simulink model "plant_test"  (R2021a)
settings: Solver=VariableStepAuto  StartTime=0.0  StopTime=10  MaxStep=0.01  RelTol=1e-3
values from neighbouring files (symbols this model uses):
  b_PID_hoist = -MEh * nh * wh    (= -542577.777778)    [Data.m]
  b_PID_trolley = MEtd*ntd*wtd    (= 540180)    [Data.m]
  bEh = 2*(bhd + bhm*ih^2)/rhd^2    (= 31004.4444444)    [Data.m]
  bEtd = (btd + btm*it^2)/rtd^2    (= 21607.2)    [Data.m]
  bt = 90    [Data.m]
  btw = 3e6    (= 3000000)    [Data.m]
  g = 9.80665    [Data.m]
  hoist_brake = readValue(uaClient,hoist_brake_node)    [Level1_OPC.m]    (also in test__TLK.m = 1; test_hoist.m = 0; test_trolley.m = 1)
  hoist_ebrake = readValue(uaClient,hoist_ebrake_node)    [Level1_OPC.m]    (also in test__TLK.m = 0; test_hoist.m = 0; test_trolley.m = 1)
  ih = 22    [Data.m]
  it = 30    [Data.m]
  Ksa_PID_hoist = -MEh * nh * wh^2    (= -1807802.81417)    [Data.m]
  Ksa_PID_trolley = MEtd*ntd*wtd^2    (= 3890592.432)    [Data.m]
  Ksia_PID_hoist = -MEh * nh * wh^3    (= -6023377.93542)    [Data.m]
  Ksia_PID_trolley = MEtd*ntd*wtd^3    (= 28021602.9322)    [Data.m]
  lh0 = 45 + 9.35    (= 54.35)    [test__TLK.m]    (also in test_hoist.m = 20; test_trolley.m = 10)
  MEh = 2*(Jhd_hEb + Jhm_hb * ih^2)/rhd^2    (= 65137.7777778)    [Data.m]
  MEtd = (Jtd + Jtm_tb*it^2)/rtd^2    (= 30000)    [Data.m]
  Ms = 15000    [Data.m]
  Mt = 30000    [Data.m]
  rhd = 0.75    [Data.m]
  rtd = 0.5    [Data.m]
  Tau_hm = 1e-3    (= 0.001)    [Data.m]
  Tau_tm = 1e-3    (= 0.001)    [Data.m]
  Th = 0    [test__TLK.m]    (also in test_hoist.m = Thm_max/5; test_trolley.m)
  Thm_max = 2.0e4    (= 20000)    [Data.m]
  trolley_brake = readValue(uaClient,trolley_brake_node)    [Level1_OPC.m]    (also in test__TLK.m = 0; test_hoist.m = 0; test_trolley.m = 0)
  Tt = 0    [test__TLK.m]    (also in test_hoist.m; test_trolley.m = Ttm_max/2)
  Ttm_max = 3.0e3    (= 3000)    [Data.m]
  xt0 = 10.55    [test__TLK.m]    (also in test_hoist.m = -20; test_trolley.m = -25)
  xtd0 = 10.55    [test__TLK.m]    (also in test_hoist.m = -20; test_trolley.m = -25)
  Yt0 = 45    [Data.m]
undefined symbols (not defined in the file or in its folder): sigbuilder_block
libraries: simulink x2
settings Model: Creator=jpss8  LastModifiedBy=jpss8

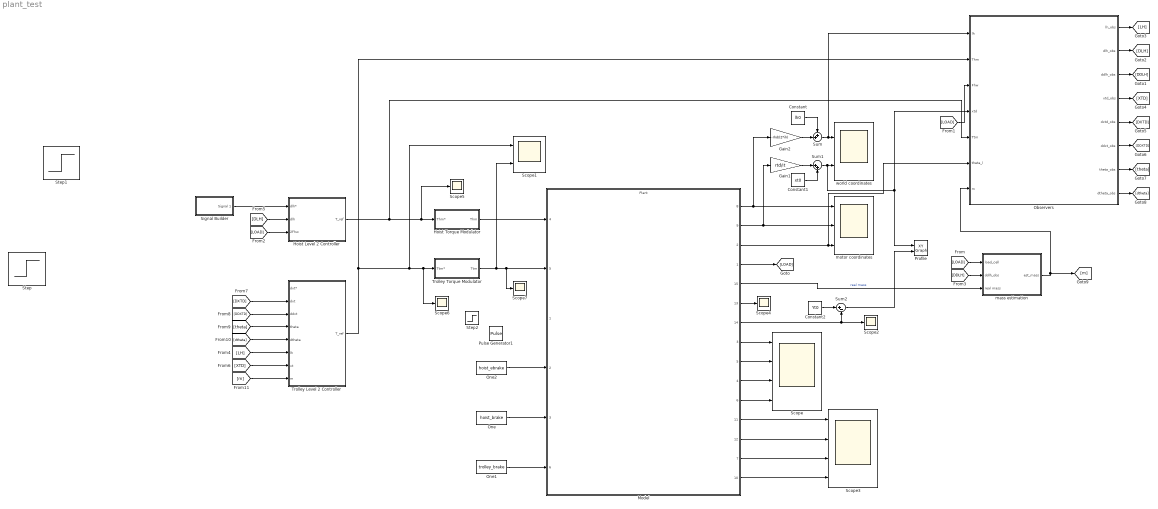
== system plant_test ==
  Constant : Constant  Value=lh0
  Constant1 : Constant  Value=xt0
  Constant2 : Constant  Value=Yt0
  Gain1 : Gain  Gain=rtd/it
  Gain2 : Gain  Gain=-rhd/(2*ih)
  Hoist Level 2 Controller : Subsystem
  Hoist Torque Modulator : Subsystem
  Model : ModelReference  ModelNameDialog=Plant.slx  SimulationMode=Normal  ModelReferenceVersion=1.173
      settings: PortSchema="{\"entries\":[{\"content\":{\"sides\":[{\"content\":{\"connectorIds\":[\"In4\",\"In5\",\"In1\",\"In2\",\"In3\",\"In6\"]},\"type\":\"ConnectorPlacement.EquallySpacedRectSide\",\"uuid\":\"c8db36dc-26e4-465b-ba81-4ad6698d5333\"},{\"content\":{\"connectorIds\":[\"Out8\",\"Out9\",\"Out2\",\"Out1\",\"Out15\",\"Out13\",\"Out14\",\"Out3\",\"Out5\",\"Out4\",\"Out6\",\"Out11\",\"Out12\",\"Out7\",\"Out10\"],\"side\":\"RIGHT\"},\"type\":\"ConnectorPlacement.EquallySpacedRectSide\",\"uuid\":\"9d1fafb8-102d-4671-8cf9-42f2986bdf69\"},{\"content\":{\"connectorIds\":[],\"side\":\"TOP\"},\"type\":\"ConnectorPlacement.EquallySpacedRectSide\",\"uuid\":\"31c48a41-488d-445d-a89d-3c2736ead4dc\"}]},\"type\":\"ConnectorPlacement.EquallySpacedConnector\",\"uuid\":\"271b3c7a-5021-4a95-89d3-3220f33b08df\"}],\"packageUris\":[\"http://schema.mathworks.com/mf0/Connector/R2020b\"],\"version\":\"1.0\"}"
  Observers : Subsystem
  One : Constant  Value=hoist_brake  OutDataTypeStr=Inherit: Inherit via back propagation
  One1 : Constant  Value=trolley_brake  OutDataTypeStr=Inherit: Inherit via back propagation
  One2 : Constant  Value=hoist_ebrake  OutDataTypeStr=Inherit: Inherit via back propagation
  Profile : simulink/Sinks/XY Graph  xmin=-30  xmax=50  ymin=-50  ymax=50  st=-1
  Pulse Generator1 : DiscretePulseGenerator  PulseType=Time based  Period=50  PulseWidth=10  PhaseDelay=1
  Scope : Scope  NumInputPorts=4
  Scope1 : Scope  NumInputPorts=2
  Scope{2,4..7} (5 alike) : Scope
  Scope3 : Scope  NumInputPorts=4
  Signal Builder : Subsystem  Tag=STV Subsys  LoadFcn=sigbuilder_block('load');  StartFcn=sigbuilder_block('start');  StopFcn=sigbuilder_block('stop');  ClipboardFcn=sigbuilder_block('clipboard');  mask(Sigbuilder block){tuvar=[0:10]}
      mask help: Simulink:masks:SigbuilderBlock_MD
      mask init:
      | if ~strcmp(get_param(bdroot(gcbh),'SimulationStatus'),'stopped') tuvar = sigbuilder_block('maskInit'); end
      settings: CopyFcn=sigbuilder_block('copy');  DeleteFcn=sigbuilder_block('delete');  ModelCloseFcn=sigbuilder_block('modelClose');  PreSaveFcn=sigbuilder_block('preSave');  PauseFcn=sigbuilder_block('pause');  ContinueFcn=sigbuilder_block('continue');  NameChangeFcn=sigbuilder_block('namechange');  OpenFcn=sigbuilder_block('open',[437.6 199.2 550.4 400 ]);  CloseFcn=sigbuilder_block('close');
      mask Display: plot(0, 0, 100, 100,[2, 2, 32, 32, 2], [68, 8, 8, 68, 68],[32, 2], [38, 38], [32, 19, 2],[53, 60, 44], [32, 17, 17, 2],[16, 16, 31, 31]);txt = getActiveGroup(gcbh);text(2, 100, txt,'verticalAlignment', 'top');
  Step : Step  After=Tt  SampleTime=0
  Step1 : Step  Time=0.5  After=Th  SampleTime=0
  Step2 : Step  Time=0.25  SampleTime=0
  Sum : Sum  Inputs=++|
  Sum1 : Sum  Inputs=|++
  Sum2 : Sum  Inputs=|+-
  Trolley Level 2 Controller : Subsystem
  Trolley Torque Modulator : Subsystem
  mass estimation : Subsystem
  motor coordinates : Scope  NumInputPorts=3
  world coordinates : Scope  NumInputPorts=2
  wires:
  Trolley Level 2 Controller/1(T_ref) -> Observers/2(Thm), Scope1/1, Scope6/1, Trolley Torque Modulator/1(Ttm*)
  Model/9 -> motor coordinates/2, Gain1/1
  Model/8 -> Gain2/1, motor coordinates/1
  Model/2 -> Observers/6(theta_l), motor coordinates/3
  Model/1 -> [LOAD]
  Model/15 -> mass estimation/3(real mass)  "real mass"
  Gain1/1 -> Sum1/1
  Gain2/1 -> Sum/2
  One1/1 -> Model/6
  One2/1 -> Model/2
  Sum/1 -> Observers/1(lh), world coordinates/1
  Constant/1 -> Sum/1
  Constant1/1 -> Sum1/2
  Model/14 -> Sum2/2, Scope2/1
  Constant2/1 -> Sum2/1
  Sum2/1 -> Profile/2
  Model/3 -> Scope/1
  Model/5 -> Scope/2
  Model/4 -> Scope/3
  Model/6 -> Scope/4
  Model/11 -> Scope3/1
  Model/12 -> Scope3/2
  Model/7 -> Scope3/3
  Model/10 -> Scope3/4
  Model/13 -> Scope4/1
  One/1 -> Model/3
  Sum1/1 -> Observers/4(xtd), Profile/1, world coordinates/2
  mass estimation/1(est_mass) -> [m], Observers/7(m)
  Observers/3(ddlh_obs) -> [DDLH]
  Hoist Torque Modulator/1(Thm) -> Model/4
  Trolley Torque Modulator/1(Ttm) -> Scope1/2, Scope7/1, Model/5
  Hoist Level 2 Controller/1(T_ref) -> Observers/5(Ttm), Scope5/1, Hoist Torque Modulator/1(Thm*)
  [LOAD] -> mass estimation/1(load_cell)
  [LOAD] -> Observers/3(Fhw)
  [LOAD] -> Hoist Level 2 Controller/3(2Fhw)
  [DDLH] -> mass estimation/2(ddlh_obs)
  Observers/2(dlh_obs) -> [DLH]
  Observers/1(lh_obs) -> [LH]
  [DLH] -> Hoist Level 2 Controller/2(dlh)
  Observers/6(ddxt_obs) -> [DDXTD]
  Observers/5(dxtd_obs) -> [DXTD]
  Observers/4(xtd_obs) -> [XTD]
  [DXTD] -> Trolley Level 2 Controller/2(dxt)
  [DDXTD] -> Trolley Level 2 Controller/3(ddxt)
  [LH] -> Trolley Level 2 Controller/6(lh)
  [XTD] -> Trolley Level 2 Controller/7(xt)
  Observers/7(theta_obs) -> [theta]
  Observers/8(dtheta_obs) -> [dtheta]
  [theta] -> Trolley Level 2 Controller/4(theta)
  [dtheta] -> Trolley Level 2 Controller/5(dtheta)
  [m] -> Trolley Level 2 Controller/8(m)
  Signal Builder/1(Signal 1) -> Hoist Level 2 Controller/1(dlh*)

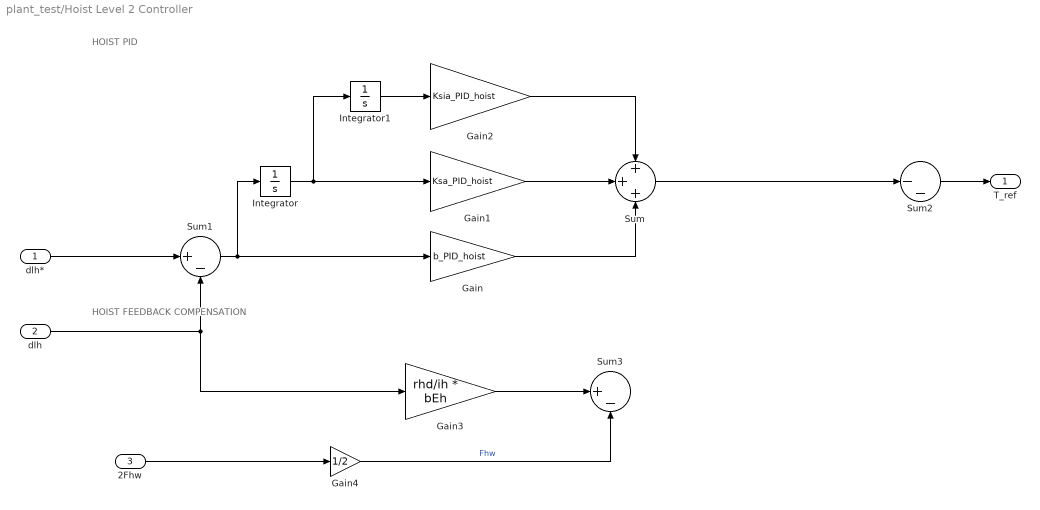
== system plant_test/Hoist Level 2 Controller ==
  note: HOIST FEEDBACK COMPENSATION
  note: HOIST PID
  dlh* : Inport
  dlh : Inport  Port=2
  2Fhw : Inport  Port=3
  Gain : Gain  Gain=b_PID_hoist
  Gain1 : Gain  Gain=Ksa_PID_hoist
  Gain2 : Gain  Gain=Ksia_PID_hoist
  Gain3 : Gain  Gain=rhd/ih * bEh
  Gain4 : Gain  Gain=1/2
  Integrator : Integrator
  Integrator1 : Integrator
  Sum : Sum  Inputs=+++
  Sum1 : Sum  Inputs=|+-
  Sum2 : Sum  Inputs=|--
  Sum3 : Sum  Inputs=|+-
  T_ref : Outport
  wires:
  Integrator/1 -> Integrator1/1, Gain1/1
  Integrator1/1 -> Gain2/1
  Gain1/1 -> Sum/2
  Gain2/1 -> Sum/1
  Gain/1 -> Sum/3
  Sum1/1 -> Gain/1, Integrator/1
  Sum/1 -> Sum2/1
  Gain3/1 -> Sum3/1
  2Fhw/1 -> Gain4/1
  Gain4/1 -> Sum3/2  "Fhw"
  dlh/1 -> Gain3/1, Sum1/2
  dlh*/1 -> Sum1/1
  Sum2/1 -> T_ref/1

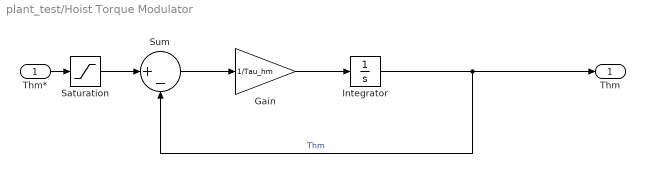
== system plant_test/Hoist Torque Modulator ==
  Thm* : Inport
  Gain : Gain  Gain=1/Tau_hm
  Integrator : Integrator
  Saturation : Saturate  UpperLimit=Thm_max  LowerLimit=-Thm_max
  Sum : Sum  Inputs=|+-
  Thm : Outport
  wires:
  Integrator/1 -> Sum/2, Thm/1  "Thm"
  Sum/1 -> Gain/1
  Gain/1 -> Integrator/1
  Thm*/1 -> Saturation/1
  Saturation/1 -> Sum/1

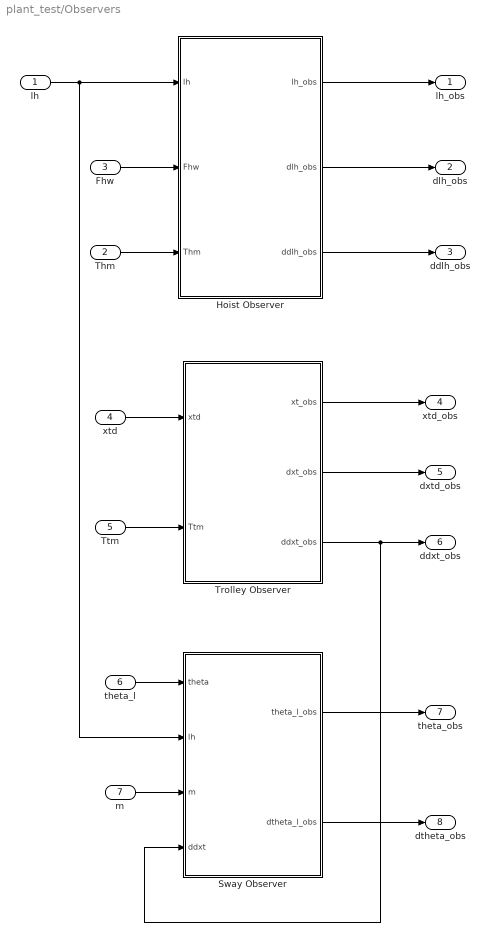
== system plant_test/Observers ==
  lh : Inport
  Thm : Inport  Port=2
  Fhw : Inport  Port=3
  xtd : Inport  Port=4
  Ttm : Inport  Port=5
  theta_l : Inport  Port=6
  m : Inport  Port=7
  Hoist Observer : Subsystem
  Sway Observer : Subsystem
  Trolley Observer : Subsystem
  lh_obs : Outport
  dlh_obs : Outport  Port=2
  ddlh_obs : Outport  Port=3
  xtd_obs : Outport  Port=4
  dxtd_obs : Outport  Port=5
  ddxt_obs : Outport  Port=6
  theta_obs : Outport  Port=7
  dtheta_obs : Outport  Port=8
  wires:
  xtd/1 -> Trolley Observer/1(xtd)
  Ttm/1 -> Trolley Observer/2(Ttm)
  Trolley Observer/1(xt_obs) -> xtd_obs/1
  Trolley Observer/2(dxt_obs) -> dxtd_obs/1
  Fhw/1 -> Hoist Observer/2(Fhw)
  Thm/1 -> Hoist Observer/3(Thm)
  Hoist Observer/1(lh_obs) -> lh_obs/1
  Hoist Observer/2(dlh_obs) -> dlh_obs/1
  theta_l/1 -> Sway Observer/1(theta)
  m/1 -> Sway Observer/3(m)
  Trolley Observer/3(ddxt_obs) -> Sway Observer/4(ddxt), ddxt_obs/1
  lh/1 -> Hoist Observer/1(lh), Sway Observer/2(lh)
  Hoist Observer/3(ddlh_obs) -> ddlh_obs/1
  Sway Observer/1(theta_l_obs) -> theta_obs/1
  Sway Observer/2(dtheta_l_obs) -> dtheta_obs/1

== system plant_test/Signal Builder ==
  Demux : Demux  Tag=STV Demux  Outputs=1
      settings: DisplayOption=none
  FromWs : FromWorkspace  Tag=STV FromWs  VariableName=tuvar
      SigBuilderData=|
      | common.afterFinalStr = 'Extrapolate'
      | common.sampleTime = 0
      | dataSet.timeRange = [0 10]
      | dataSet.name = 'Group 1'
      | sbobj.Groups.Name = 'Group 1'
      | sbobj.Groups.Signals.Name = 'Signal 1'
      | sbobj.Groups.Signals.XData = [0 2 8 10]
      | sbobj.Groups.Signals.YData = [0 3 3 0]
  Signal 1 : Outport  Tag=STV Outport
  wires:
  Demux/1 -> Signal 1/1
  FromWs/1 -> Demux/1

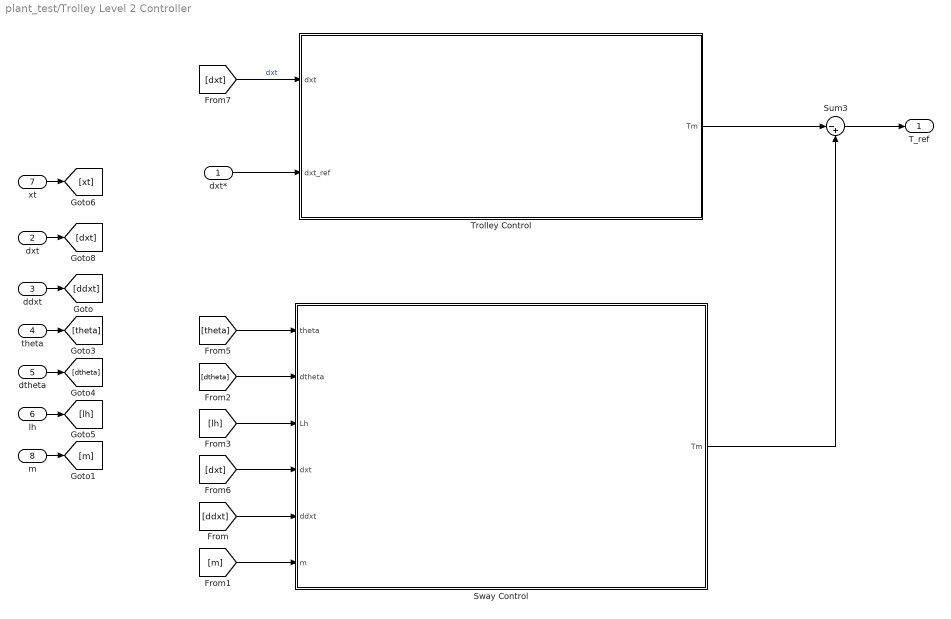
== system plant_test/Trolley Level 2 Controller ==
  dxt* : Inport
  dxt : Inport  Port=2
  ddxt : Inport  Port=3
  theta : Inport  Port=4
  dtheta : Inport  Port=5
  lh : Inport  Port=6
  xt : Inport  Port=7
  m : Inport  Port=8
  Sum3 : Sum  Inputs=|-+
  Sway Control : Subsystem
  Trolley Control : Subsystem
  T_ref : Outport
  wires:
  ddxt/1 -> [ddxt]
  lh/1 -> [lh]
  dtheta/1 -> [dtheta]
  theta/1 -> [theta]
  dxt/1 -> [dxt]
  [dxt] -> Trolley Control/1(dxt)  "dxt"
  Sum3/1 -> T_ref/1
  [lh] -> Sway Control/3(Lh)
  [dxt] -> Sway Control/4(dxt)
  xt/1 -> [xt]
  dxt*/1 -> Trolley Control/2(dxt_ref)
  Sway Control/1(Tm) -> Sum3/2
  [theta] -> Sway Control/1(theta)
  [dtheta] -> Sway Control/2(dtheta)
  Trolley Control/1(Tm) -> Sum3/1
  [ddxt] -> Sway Control/5(ddxt)
  [m] -> Sway Control/6(m)
  m/1 -> [m]

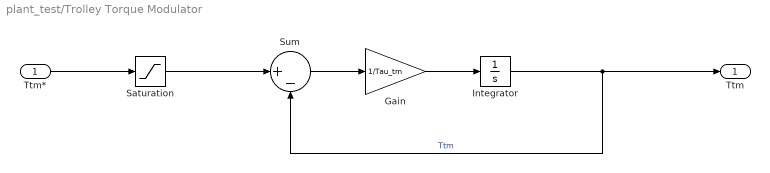
== system plant_test/Trolley Torque Modulator ==
  Ttm* : Inport
  Gain : Gain  Gain=1/Tau_tm
  Integrator : Integrator
  Saturation : Saturate  UpperLimit=Ttm_max  LowerLimit=-Ttm_max
  Sum : Sum  Inputs=|+-
  Ttm : Outport
  wires:
  Gain/1 -> Integrator/1
  Sum/1 -> Gain/1
  Integrator/1 -> Ttm/1, Sum/2  "Ttm"
  Ttm*/1 -> Saturation/1
  Saturation/1 -> Sum/1

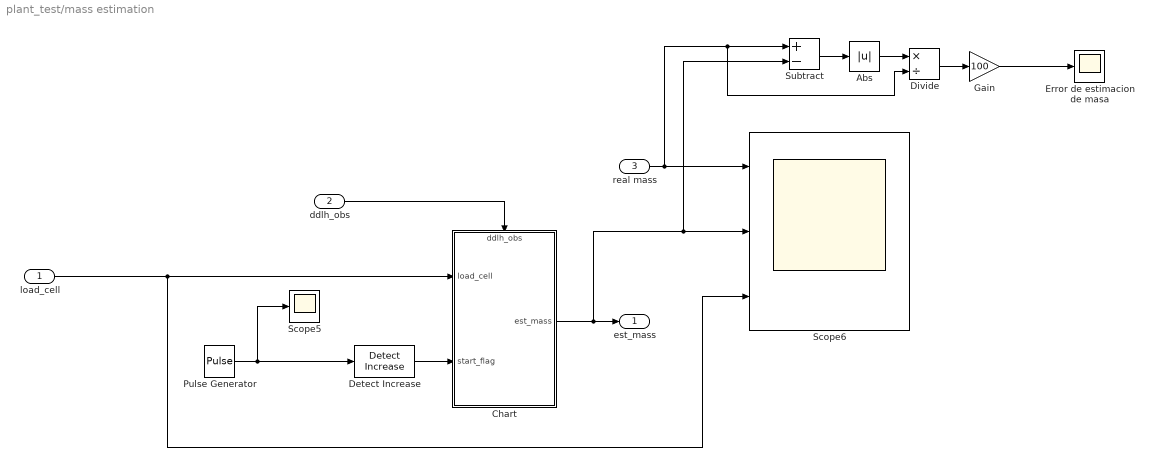
== system plant_test/mass estimation ==
  load_cell : Inport
  ddlh_obs : Inport  Port=2
  real mass : Inport  Port=3
  Abs : Abs
  Chart : Stateflow chart  TreatAsAtomicUnit=on
      settings: PortSchema="{\"entries\":[{\"content\":{\"sides\":[{\"content\":{\"connectorIds\":[\"In2\",\"In3\"]},\"type\":\"ConnectorPlacement.EquallySpacedRectSide\",\"uuid\":\"44794d8c-8d17-4178-a01f-d04d4719ed54\"},{\"content\":{\"connectorIds\":[\"Out1\"],\"side\":\"RIGHT\"},\"type\":\"ConnectorPlacement.EquallySpacedRectSide\",\"uuid\":\"4fbe92f0-b9dd-4e22-a980-5654a9e61553\"},{\"content\":{\"connectorIds\":[\"In1\"],\"side\":\"TOP\"},\"type\":\"ConnectorPlacement.EquallySpacedRectSide\",\"uuid\":\"c0e4bb71-f4b3-4ee0-bf7e-beab745a0d9c\"}]},\"type\":\"ConnectorPlacement.EquallySpacedConnector\",\"uuid\":\"86c94122-6cae-4719-99cd-dfe2bbeee74d\"}],\"packageUris\":[\"http://schema.mathworks.com/mf0/Connector/R2020b\"],\"version\":\"1.0\"}"
  Detect Increase : simulink/Logic and Bit Operations/Detect Increase  vinit=0.0  OutDataTypeStr=boolean
  Divide : Product  Inputs=*/
  Error de estimacion de masa : Scope
  Gain : Gain  Gain=100
  Pulse Generator : DiscretePulseGenerator  PulseType=Time based  Period=50  PulseWidth=2  PhaseDelay=3
  Scope5 : Scope
  Scope6 : Scope  NumInputPorts=3
  Subtract : Sum  Inputs=+-
  est_mass : Outport
  wires:
  load_cell/1 -> Chart/2(load_cell), Scope6/3
  Detect Increase/1 -> Chart/3(start_flag)
  Pulse Generator/1 -> Scope5/1, Detect Increase/1
  Chart/1(est_mass) -> est_mass/1, Subtract/2, Scope6/2
  real mass/1 -> Divide/2, Subtract/1, Scope6/1
  Subtract/1 -> Abs/1
  Abs/1 -> Divide/1
  Divide/1 -> Gain/1
  Gain/1 -> Error de estimacion de masa/1
  ddlh_obs/1 -> Chart/1(ddlh_obs)

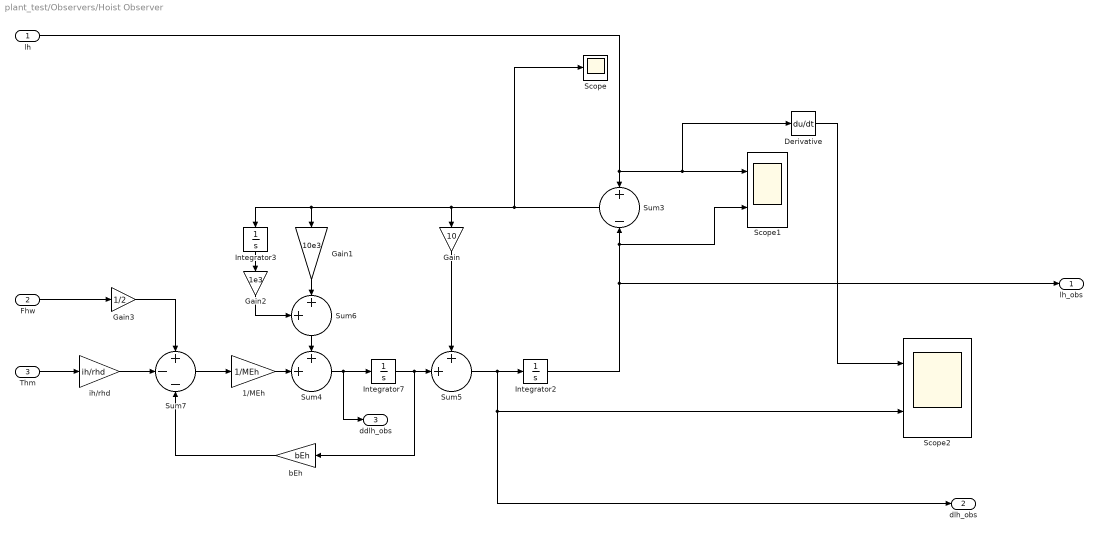
== system plant_test/Observers/Hoist Observer ==
  lh : Inport
  Fhw : Inport  Port=2
  Thm : Inport  Port=3
  1/MEh : Gain  Gain=1/MEh
  Derivative : Derivative
  Gain : Gain  Gain=10
  Gain1 : Gain  Gain=10e3
  Gain2 : Gain  Gain=1e3
  Gain3 : Gain  Gain=1/2
  Integrator2 : Integrator  InitialCondition=lh0
  Integrator3 : Integrator
  Integrator7 : Integrator
  Scope : Scope
  Scope1 : Scope  NumInputPorts=2
  Scope2 : Scope  NumInputPorts=2
  Sum3 : Sum  Inputs=+|-
  Sum4 : Sum  Inputs=++|
  Sum5 : Sum  Inputs=++|
  Sum6 : Sum  Inputs=++|
  Sum7 : Sum  Inputs=+--
  bEh : Gain  Gain=bEh
  ih/rhd : Gain  Gain=ih/rhd
  lh_obs : Outport
  dlh_obs : Outport  Port=2
  ddlh_obs : Outport  Port=3
  wires:
  Sum5/1 -> dlh_obs/1, Scope2/2, Integrator2/1
  lh/1 -> Sum3/1, Derivative/1, Scope1/1
  Gain1/1 -> Sum6/2
  Gain3/1 -> Sum7/1
  Integrator3/1 -> Gain2/1
  bEh/1 -> Sum7/3
  Sum3/1 -> Scope/1, Gain/1, Integrator3/1, Gain1/1
  ih/rhd/1 -> Sum7/2
  Sum7/1 -> 1/MEh/1
  Sum4/1 -> ddlh_obs/1, Integrator7/1
  Gain/1 -> Sum5/1
  Integrator2/1 -> lh_obs/1, Scope1/2, Sum3/2
  Sum6/1 -> Sum4/1
  Integrator7/1 -> bEh/1, Sum5/2
  1/MEh/1 -> Sum4/2
  Derivative/1 -> Scope2/1
  Thm/1 -> ih/rhd/1
  Fhw/1 -> Gain3/1
  Gain2/1 -> Sum6/1

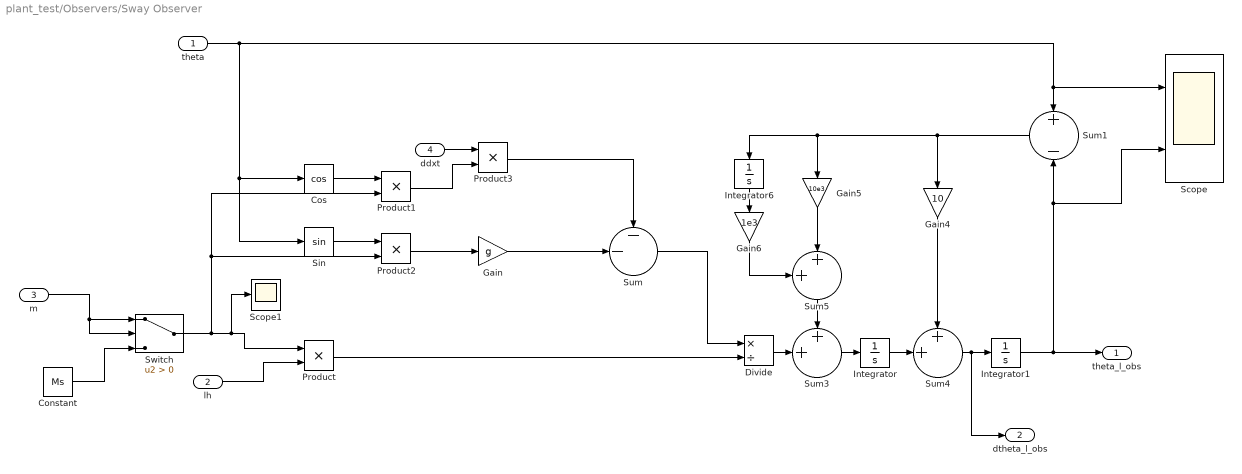
== system plant_test/Observers/Sway Observer ==
  theta : Inport
  lh : Inport  Port=2
  m : Inport  Port=3
  ddxt : Inport  Port=4
  Constant : Constant  Value=Ms
  Cos : Trigonometry  Operator=cos
  Divide : Product  Inputs=*/
  Gain : Gain  Gain=g
  Gain4 : Gain  Gain=10
  Gain5 : Gain  Gain=10e3
  Gain6 : Gain  Gain=1e3
  Integrator : Integrator
  Integrator1 : Integrator
  Integrator6 : Integrator
  Product{,1..3} (4 alike) : Product
  Scope : Scope  NumInputPorts=2
  Scope1 : Scope
  Sin : Trigonometry
  Sum : Sum  Inputs=--|
  Sum1 : Sum  Inputs=+|-
  Sum3 : Sum  Inputs=++|
  Sum4 : Sum  Inputs=++|
  Sum5 : Sum  Inputs=++|
  Switch : Switch  Criteria=u2 > Threshold
  theta_l_obs : Outport
  dtheta_l_obs : Outport  Port=2
  wires:
  Product/1 -> Divide/2
  theta/1 -> Sin/1, Cos/1, Scope/1, Sum1/1
  lh/1 -> Product/2
  Divide/1 -> Sum3/2
  Product3/1 -> Sum/1
  Cos/1 -> Product1/1
  Sin/1 -> Product2/1
  Product2/1 -> Gain/1
  Gain/1 -> Sum/2
  Product1/1 -> Product3/2
  ddxt/1 -> Product3/1
  Sum/1 -> Divide/1
  Integrator1/1 -> theta_l_obs/1, Scope/2, Sum1/2
  Sum1/1 -> Gain5/1, Integrator6/1, Gain4/1
  Gain5/1 -> Sum5/2
  Integrator6/1 -> Gain6/1
  Gain6/1 -> Sum5/1
  Sum3/1 -> Integrator/1
  Sum4/1 -> dtheta_l_obs/1, Integrator1/1
  Sum5/1 -> Sum3/1
  Gain4/1 -> Sum4/1
  Integrator/1 -> Sum4/2
  m/1 -> Switch/2, Switch/1
  Switch/1 -> Scope1/1, Product/1, Product1/2, Product2/2
  Constant/1 -> Switch/3

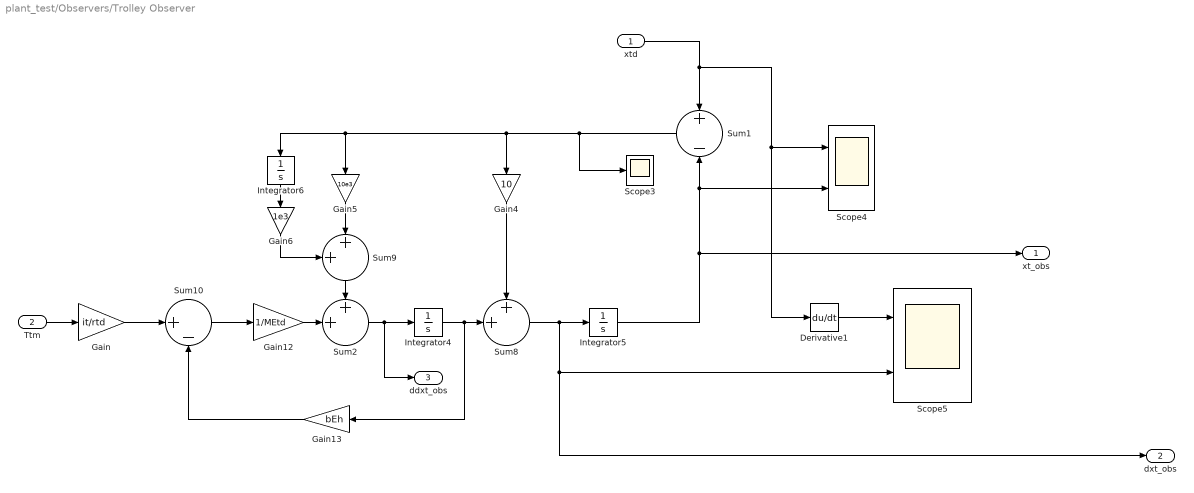
== system plant_test/Observers/Trolley Observer ==
  xtd : Inport
  Ttm : Inport  Port=2
  Derivative1 : Derivative
  Gain : Gain  Gain=it/rtd
  Gain12 : Gain  Gain=1/MEtd
  Gain13 : Gain  Gain=bEh
  Gain4 : Gain  Gain=10
  Gain5 : Gain  Gain=10e3
  Gain6 : Gain  Gain=1e3
  Integrator4 : Integrator
  Integrator5 : Integrator  InitialCondition=xtd0
  Integrator6 : Integrator
  Scope3 : Scope
  Scope4 : Scope  NumInputPorts=2
  Scope5 : Scope  NumInputPorts=2
  Sum1 : Sum  Inputs=+|-
  Sum10 : Sum  Inputs=|+-
  Sum2 : Sum  Inputs=++|
  Sum8 : Sum  Inputs=++|
  Sum9 : Sum  Inputs=++|
  xt_obs : Outport
  dxt_obs : Outport  Port=2
  ddxt_obs : Outport  Port=3
  wires:
  Sum2/1 -> ddxt_obs/1, Integrator4/1
  Sum8/1 -> Integrator5/1, dxt_obs/1, Scope5/2
  Gain4/1 -> Sum8/1
  Integrator4/1 -> Sum8/2, Gain13/1
  Sum1/1 -> Gain5/1, Integrator6/1, Gain4/1, Scope3/1
  Derivative1/1 -> Scope5/1
  Integrator5/1 -> xt_obs/1, Sum1/2, Scope4/2
  xtd/1 -> Sum1/1, Derivative1/1, Scope4/1
  Gain12/1 -> Sum2/2
  Gain5/1 -> Sum9/2
  Gain/1 -> Sum10/1
  Gain13/1 -> Sum10/2
  Sum10/1 -> Gain12/1
  Gain6/1 -> Sum9/1
  Sum9/1 -> Sum2/1
  Integrator6/1 -> Gain6/1
  Ttm/1 -> Gain/1

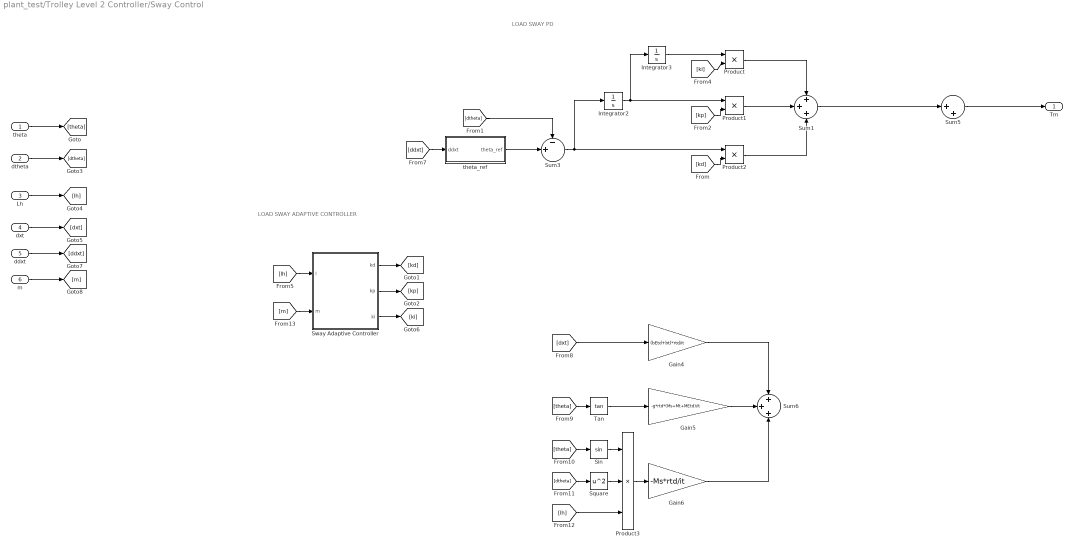
== system plant_test/Trolley Level 2 Controller/Sway Control ==
  note: LOAD SWAY ADAPTIVE CONTROLLER
  note: LOAD SWAY PD
  theta : Inport
  dtheta : Inport  Port=2
  Lh : Inport  Port=3
  dxt : Inport  Port=4
  ddxt : Inport  Port=5
  m : Inport  Port=6
  Gain4 : Gain  Gain=(bEtd+bt)*rtd/it
  Gain5 : Gain  Gain=-g*rtd*(Ms+Mt+MEtd)/it
  Gain6 : Gain  Gain=-Ms*rtd/it
  Integrator2 : Integrator
  Integrator3 : Integrator
  Product : Product
  Product1 : Product
  Product2 : Product
  Product3 : Product  Inputs=3
  Sin : Trigonometry
  Square : Math  Operator=square  SaturateOnIntegerOverflow=on
  Sum1 : Sum  Inputs=+++
  Sum3 : Sum  Inputs=-+|
  Sum5 : Sum  Inputs=|++
  Sum6 : Sum  Inputs=+++
  Sway Adaptive Controller : Subsystem
  Tan : Trigonometry  Operator=tan
  theta_ref : Subsystem
  Tm : Outport
  wires:
  Sway Adaptive Controller/3(ki) -> [ki]
  Sway Adaptive Controller/2(kp) -> [kp]
  Integrator2/1 -> Integrator3/1, Product1/1
  [dxt] -> Gain4/1
  [theta] -> Sin/1
  Product1/1 -> Sum1/2
  Integrator3/1 -> Product/1
  [kp] -> Product1/2
  [dtheta] -> Sum3/1
  Sway Adaptive Controller/1(kd) -> [kd]
  Sum3/1 -> Product2/1, Integrator2/1
  [lh] -> Sway Adaptive Controller/1(l)
  Sin/1 -> Product3/1
  Product3/1 -> Gain6/1
  Product2/1 -> Sum1/3
  Sum5/1 -> Tm/1
  Product/1 -> Sum1/1
  Sum1/1 -> Sum5/1
  [ki] -> Product/2
  theta_ref/1(theta_ref) -> Sum3/2
  [theta] -> Tan/1
  Gain4/1 -> Sum6/1
  [kd] -> Product2/2
  Square/1 -> Product3/2
  Gain5/1 -> Sum6/2
  Tan/1 -> Gain5/1
  [dtheta] -> Square/1
  [lh] -> Product3/3
  Gain6/1 -> Sum6/3
  theta/1 -> [theta]
  dtheta/1 -> [dtheta]
  Lh/1 -> [lh]
  dxt/1 -> [dxt]
  ddxt/1 -> [ddxt]
  [ddxt] -> theta_ref/1(ddxt)
  m/1 -> [m]
  [m] -> Sway Adaptive Controller/2(m)

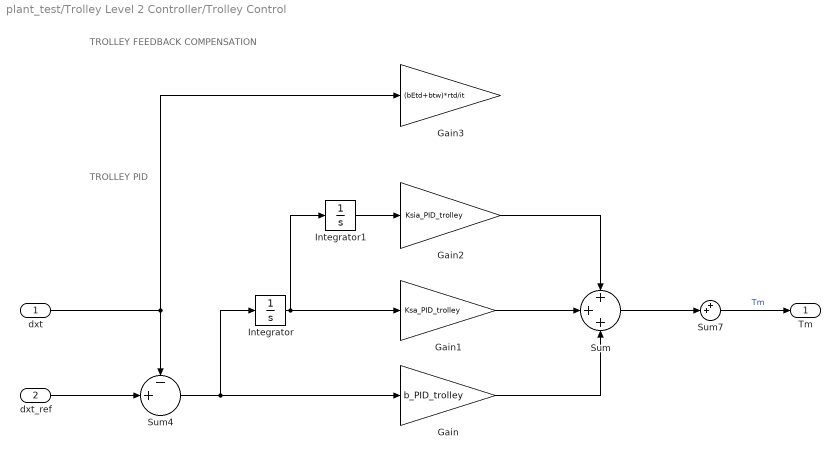
== system plant_test/Trolley Level 2 Controller/Trolley Control ==
  note: TROLLEY FEEDBACK COMPENSATION
  note: TROLLEY PID
  dxt : Inport
  dxt_ref : Inport  Port=2
  Gain : Gain  Gain=b_PID_trolley
  Gain1 : Gain  Gain=Ksa_PID_trolley
  Gain2 : Gain  Gain=Ksia_PID_trolley
  Gain3 : Gain  Gain=(bEtd+btw)*rtd/it
  Integrator : Integrator
  Integrator1 : Integrator
  Sum : Sum  Inputs=+++
  Sum4 : Sum  Inputs=-+|
  Sum7 : Sum  Inputs=++|
  Tm : Outport
  wires:
  dxt/1 -> Sum4/1, Gain3/1
  Gain2/1 -> Sum/1
  Gain/1 -> Sum/3
  Integrator1/1 -> Gain2/1
  Sum7/1 -> Tm/1  "Tm"
  Gain1/1 -> Sum/2
  Sum/1 -> Sum7/2
  dxt_ref/1 -> Sum4/2
  Sum4/1 -> Integrator/1, Gain/1
  Integrator/1 -> Integrator1/1, Gain1/1

== system plant_test/Trolley Level 2 Controller/Sway Control/Sway Adaptive Controller ==
  l : Inport
  m : Inport  Port=2
  MATLAB Function : MATLAB Function  TreatAsAtomicUnit=on
  kd : Outport
  kp : Outport  Port=2
  ki : Outport  Port=3
  wires:
  MATLAB Function/2(kp) -> ?
  MATLAB Function/1(kd) -> ?
  l/1 -> ?
  MATLAB Function/3(ki) -> ?
  m/1 -> ?

== system plant_test/Trolley Level 2 Controller/Sway Control/theta_ref ==
  ddxt : Inport
  Gain : Gain  Gain=-10
  theta_ref : Outport
  wires:
  ddxt/1 -> Gain/1
  Gain/1 -> theta_ref/1

== matlab function plant_test/Trolley Level 2 Controller/Sway Control/Sway Adaptive Controller/MATLAB Function ==
  data: lh input; ml input; kd output; kp output; ki output
function [kd, kp, ki] = get_sway_adaptive_gains(lh, ml)
g=9.81;
Mt = 30000;

aux = (Mt+ml)*lh;

wn = sqrt(Mt*g/aux);

g=9.81;
Mt = 30000;
kd = -lh + ( (Mt*g)/((wn)*(ml+Mt)) ) ;
kp = 2*wn*(lh + kd);
ki = 0;

end

== stateflow chart plant_test/mass estimation/Chart ==
  state Standby
    entry:
    end_flag = 0;
    sum = 0;
    i = 0;
    tol = 1e-2;
    prev_mass = 0;
    diff = 1e5; %big number
  state CalculateMass
    measurement = load_cell;
    acc = ddlh_obs;
    state Estimation
      during:
      sum = sum +  measurement;
      i = i + 1;
      force_avg = sum/i;
      mass = force_avg/(g-acc);
      diff = abs(mass - prev_mass)/mass;
      prev_mass = mass;
    state StableValue
      entry:
      est_mass = mass;
      end_flag = 1;
    (default) -> Estimation
    Estimation -> StableValue : [diff<tol]
  (default) -> Standby
  Standby -> CalculateMass : [start_flag]
  CalculateMass -> Standby : [end_flag]
  data: ddlh_obs input; load_cell input; start_flag input; end_flag local; i local; measurement local; sum local; g parameter double; force_avg local; diff local; tol local; prev_mass local; est_mass output; mass local; acc local
